simulink model "understandingof_cotangentwave"  (R2024b)
settings: Solver=VariableStepAuto  StartTime=0.0  StopTime=25  MaxStep=0.001  RelTol=1e-3
settings Model: Creator=admin  LastModifiedBy=admin

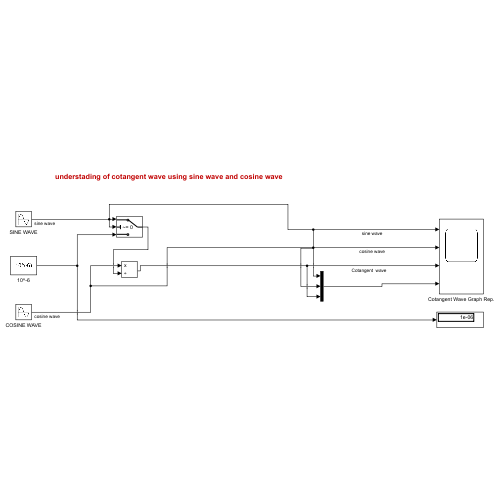
[thumbnail: Simulink's stored preview of the top-level diagram]
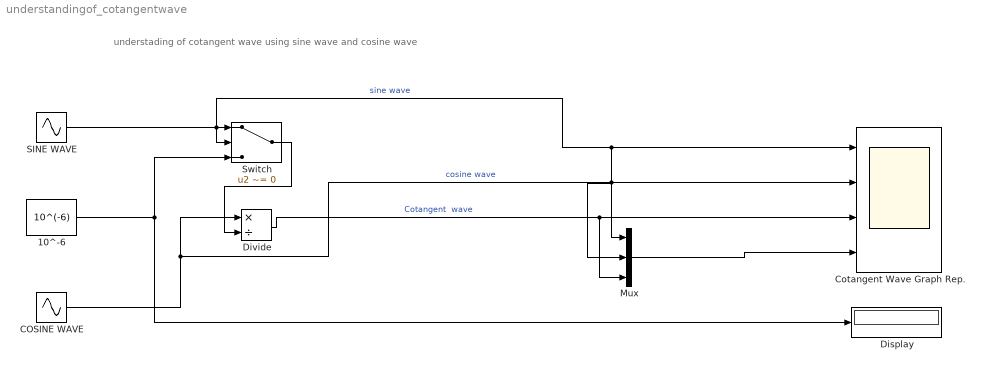
== system understandingof_cotangentwave ==
  note: understading of cotangent wave using sine wave and cosine wave
  10^-6 : Constant  Value=10^(-6)
  COSINE WAVE : Sin  Phase=pi/2  SampleTime=0
  Cotangent Wave Graph Rep. : Scope  NumInputPorts=4
  Display : Display
  Divide : Product  Inputs=*/
  Mux : Mux  Inputs=3
  SINE WAVE : Sin  SampleTime=0
  Switch : Switch  Criteria=u2 ~= 0  SaturateOnIntegerOverflow=off  InputSameDT=off
  wires:
  10^-6/1 -> Display/1, Switch/3
  SINE WAVE/1 -> Switch/2, Switch/1, Mux/1, Cotangent Wave Graph Rep./1  "sine wave"
  COSINE WAVE/1 -> Mux/2, Cotangent Wave Graph Rep./2, Divide/1  "cosine wave"
  Switch/1 -> Divide/2
  Divide/1 -> Cotangent Wave Graph Rep./3, Mux/3  "Cotangent  wave"
  Mux/1 -> Cotangent Wave Graph Rep./4
